simulink model "Mdl_LPVOL"  (R2021b)
settings: Solver=FixedStepAuto  StartTime=0.0  StopTime=10.0  FixedStep=DT  RelTol=1e-3
values from neighbouring files (symbols this model uses):
  OutList = <binary blob, 363 chars, not shown>    [DD_LPV.sldd]
undefined symbols (not defined in the file or in its folder): strmatch, sys12d_w
libraries: cstblocks x1
settings Model: DataDictionary=DD_LPV.sldd  Creator=ditt_aj  LastModifiedBy=ditt_aj
settings SolverCC: AlgebraicLoopSolver=TrustRegion
settings DebuggingCC: SFMachineParentedDataDiag=warning
settings SFSimCC: CustomCodeUndefinedFunction=UseInterfaceOnly

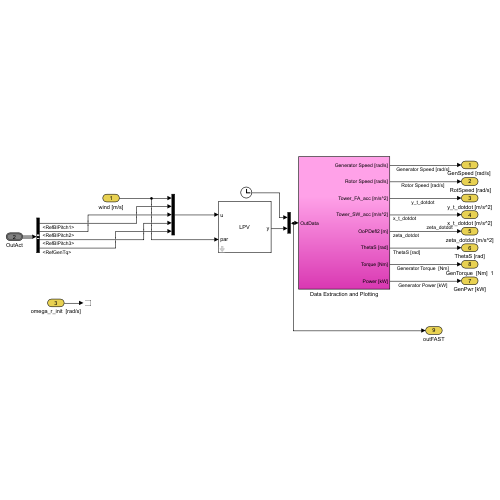
[thumbnail: Simulink's stored preview of the top-level diagram]
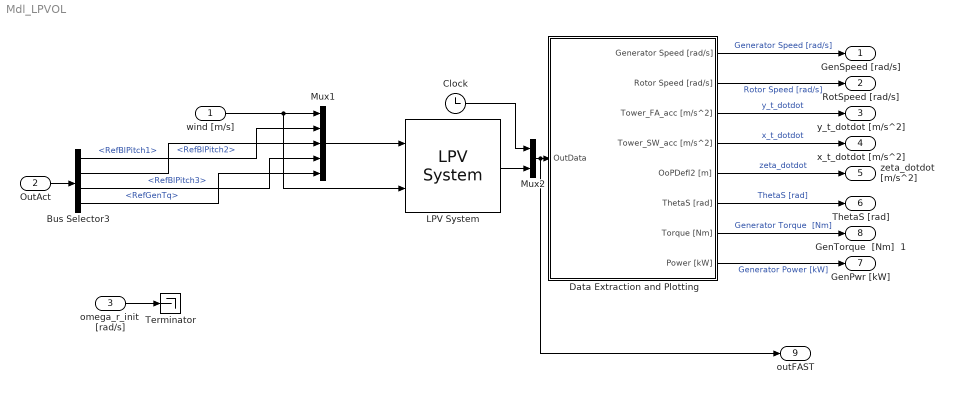
== system Mdl_LPVOL ==
  wind [m/s] : Inport
  OutAct : Inport  Port=2  OutDataTypeStr=Bus: slBus2
  omega_r_init  [rad/s] : Inport  Port=3
  Bus Selector3 : BusSelector  OutputSignals=RefBlPitch1,RefBlPitch2,RefBlPitch3,RefGenTq
  Clock : Clock
  Data Extraction and Plotting : Subsystem
  LPV System : cstblocks/Linear Parameter Varying/LPV System  sys=sysd  x0=x0  uOffset=uoff  yOffset=yoff  xOffset=xoff  opEquilOption=on  dxOffset=0  sysFixedOption=Use the first model in state-space array  sysFixed=sys12d_w(:,:,4)  AFixed=false  BFixed=false  CFixed=false  DFixed=false  uDelayFixed=false  yDelayFixed=false  iDelayFixed=false  IMethod=Nearest  EMethod=Clip  IndexSearch=Binary search  IndexBegin=on  OutputX=off  OutputXdot=off  OutputLTI=off  OutputOP=off  DataType=double  SimMode=Interpreted execution  InitBufferSize=1024  FixedBuffer=off
      settings: SourceProductBaseCode=CT
  Mux1 : Mux  Inputs=5
  Mux2 : Mux  Inputs=2
  Terminator : Terminator
  "GenSpeed [rad/s] " : Outport  VectorParamsAs1DForOutWhenUnconnected=off
  " RotSpeed [rad/s]" : Outport  Port=2  VectorParamsAs1DForOutWhenUnconnected=off
  y_t_dotdot [m/s^2] : Outport  Port=3  VectorParamsAs1DForOutWhenUnconnected=off
  x_t_dotdot [m/s^2] : Outport  Port=4  VectorParamsAs1DForOutWhenUnconnected=off
  zeta_dotdot [m/s^2] : Outport  Port=5  VectorParamsAs1DForOutWhenUnconnected=off
  ThetaS [rad] : Outport  Port=6  VectorParamsAs1DForOutWhenUnconnected=off
  GenPwr [kW] : Outport  Port=7  VectorParamsAs1DForOutWhenUnconnected=off
  GenTorque  [Nm]  1 : Outport  Port=8  VectorParamsAs1DForOutWhenUnconnected=off
  outFAST : Outport  Port=9  VectorParamsAs1DForOutWhenUnconnected=off
  wires:
  wind [m/s]/1 -> LPV System/2, Mux1/1
  Mux1/1 -> LPV System/1
  Clock/1 -> Mux2/1
  LPV System/1 -> Mux2/2
  Mux2/1 -> outFAST/1, Data Extraction and Plotting/1(OutData)
  Data Extraction and Plotting/6(ThetaS [rad]) -> ThetaS [rad]/1  "ThetaS [rad]"
  Data Extraction and Plotting/7(Torque [Nm]) -> GenTorque  [Nm]  1/1  "Generator Torque  [Nm]"
  Data Extraction and Plotting/8(Power [kW]) -> GenPwr [kW]/1  "Generator Power [kW]"
  Data Extraction and Plotting/5(OoPDefl2 [m]) -> zeta_dotdot [m/s^2]/1  "zeta_dotdot"
  Data Extraction and Plotting/4(Tower_SW_acc [m/s^2]) -> x_t_dotdot [m/s^2]/1  "x_t_dotdot"
  Data Extraction and Plotting/3(Tower_FA_acc [m/s^2]) -> y_t_dotdot [m/s^2]/1  "y_t_dotdot"
  Data Extraction and Plotting/1(Generator Speed [rad/s]) -> "GenSpeed [rad/s] "/1  "Generator Speed [rad/s]"
  Data Extraction and Plotting/2(Rotor Speed [rad/s]) -> " RotSpeed [rad/s]"/1  "Rotor Speed [rad/s]"
  omega_r_init  [rad/s]/1 -> Terminator/1
  OutAct/1 -> Bus Selector3/1
  Bus Selector3/1 -> Mux1/2  "<RefBlPitch1>"
  Bus Selector3/2 -> Mux1/3  "<RefBlPitch2>"
  Bus Selector3/3 -> Mux1/4  "<RefBlPitch3>"
  Bus Selector3/4 -> Mux1/5  "<RefGenTq>"

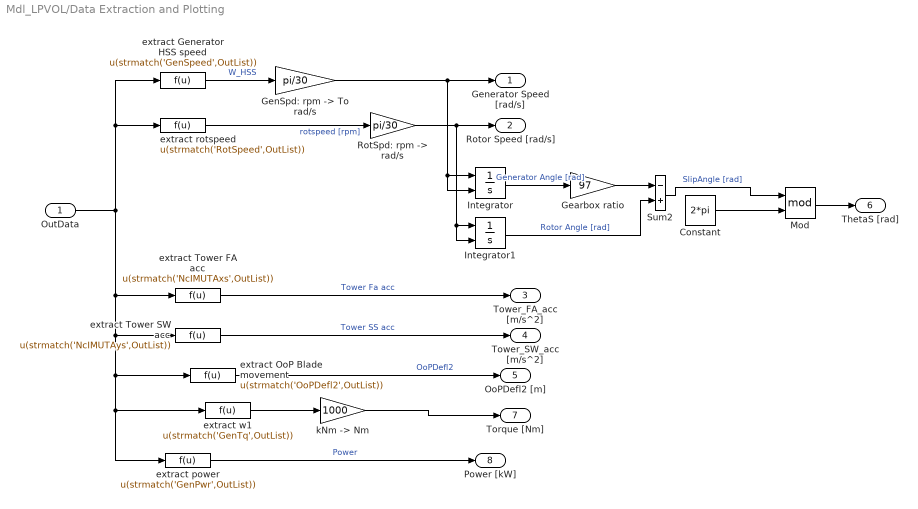
== system Mdl_LPVOL/Data Extraction and Plotting ==
  OutData : Inport
  Constant : Constant  Value=2*pi
  Gearbox ratio : Gain  Gain=97
  "GenSpd: rpm -> To rad/s" : Gain  Gain=pi/30
  Integrator : Integrator  InitialConditionSource=external
  Integrator1 : Integrator  InitialConditionSource=external
  Mod : Math  Operator=mod  SaturateOnIntegerOverflow=on
  "RotSpd: rpm -> rad/s" : Gain  Gain=pi/30
  Sum2 : Sum  Inputs=-+
  extract Generator HSS speed : Fcn  Expr=u(strmatch('GenSpeed',OutList))
  extract OoP Blade movement : Fcn  Expr=u(strmatch('OoPDefl2',OutList))
  extract Tower FA acc : Fcn  Expr=u(strmatch('NcIMUTAxs',OutList))
  extract Tower SW acc : Fcn  Expr=u(strmatch('NcIMUTAys',OutList))
  extract power : Fcn  Expr=u(strmatch('GenPwr',OutList))
  extract rotspeed : Fcn  Expr=u(strmatch('RotSpeed',OutList))
  extract w1 : Fcn  Expr=u(strmatch('GenTq',OutList))
  "kNm -> Nm" : Gain  Gain=1000
  Generator Speed [rad/s] : Outport  VectorParamsAs1DForOutWhenUnconnected=off
  Rotor Speed [rad/s] : Outport  Port=2  VectorParamsAs1DForOutWhenUnconnected=off
  Tower_FA_acc [m/s^2] : Outport  Port=3  VectorParamsAs1DForOutWhenUnconnected=off
  Tower_SW_acc [m/s^2] : Outport  Port=4  VectorParamsAs1DForOutWhenUnconnected=off
  OoPDefl2 [m] : Outport  Port=5  VectorParamsAs1DForOutWhenUnconnected=off
  ThetaS [rad] : Outport  Port=6  VectorParamsAs1DForOutWhenUnconnected=off
  Torque [Nm] : Outport  Port=7  VectorParamsAs1DForOutWhenUnconnected=off
  Power [kW] : Outport  Port=8  VectorParamsAs1DForOutWhenUnconnected=off
  wires:
  extract rotspeed/1 -> "RotSpd: rpm -> rad/s"/1  "rotspeed [rpm]"
  extract power/1 -> Power [kW]/1  "Power"
  extract Tower FA acc/1 -> Tower_FA_acc [m/s^2]/1  "Tower Fa acc"
  extract Tower SW acc/1 -> Tower_SW_acc [m/s^2]/1  "Tower SS acc"
  extract w1/1 -> "kNm -> Nm"/1
  "kNm -> Nm"/1 -> Torque [Nm]/1
  "RotSpd: rpm -> rad/s"/1 -> Integrator1/2, Integrator1/1, Rotor Speed [rad/s]/1
  "GenSpd: rpm -> To rad/s"/1 -> Integrator/2, Integrator/1, Generator Speed [rad/s]/1
  extract Generator HSS speed/1 -> "GenSpd: rpm -> To rad/s"/1  "W_HSS"
  extract OoP Blade movement/1 -> OoPDefl2 [m]/1  "OoPDefl2"
  OutData/1 -> extract power/1, extract w1/1, extract OoP Blade movement/1, extract Tower SW acc/1, extract Tower FA acc/1, extract Generator HSS speed/1, extract rotspeed/1
  Integrator/1 -> Gearbox ratio/1  "Generator Angle [rad]"
  Integrator1/1 -> Sum2/2  "Rotor Angle [rad]"
  Sum2/1 -> Mod/1  "SlipAngle [rad]"
  Constant/1 -> Mod/2
  Mod/1 -> ThetaS [rad]/1
  Gearbox ratio/1 -> Sum2/1
